simulink model "Exp_MLegMotor_PD_Sine"  (R2014b)
settings: Solver=ode1  StartTime=0.0  StopTime=Inf  FixedStep=0.001  RelTol=1e-3
PostLoadFcn:
  | , if any(exist('dsrtsu_mdlpostloadfcn', 'file') == [2, 3, 6]), try dsrtsu_mdlpostloadfcn('Execute', bdroot); catch fprintf('Error in PostLoadFcn (dsrtsu_mdlpostloadfcn) for model "%s":\n %s\n', bdroot, lasterr); end, end,
values from neighbouring files (symbols this model uses):
  coulomb_feedforward_coeff = 0    [init.m]
  enable_motor = 0    [init.m]
  filter_switch = 1    [init.m]
  Kd = 0.1    [init.m]
  Kp = 15    [init.m]
  motor_cutoff_angle = 70 * pi/180    (= 1.2217304764)    [init.m]
  motor_direction = -1    [init.m]
  pos_weight_1 = 0    [init.m]
  pos_weight_2 = 0    [init.m]
  ref_amplitude = 4    [init.m]
  ref_frequency = 0.5    [init.m]
  savgol_k = 2    [init.m]
  savgol_m = 150    [init.m]
  Ts = 0.001    [init.m]
undefined symbols (not defined in the file): max_ddphi, max_dphi, red_alpha, red_lambda
libraries: rtilib1103 x3, simulink x2, simulink_extras x1
settings Model: DSRTSU_INTERNAL_RTI_VER=450  DSRTSU_INTERNAL_RTI_TYPE=rti1103  DSRTSU_INTERNAL_RTIFPGA=40  TunableVars=Kd,Kp,coulomb_feedforward_coeff,enable_motor,filter_switch,motor_cutoff_angle,pos_weight_1,pos_weight_2,ref_amplitude,ref_frequency  TunableVarsStorageClass=Auto,Auto,Auto,Auto,Auto,Auto,Auto,Auto,Auto,Auto  TunableVarsTypeQualifier=,,,,,,,,,  BufferReuse=off  Creator=robotuser  LastModifiedBy=robotuser
settings OptimizationCC: BlockReduction=off  InlineParams=on  OptimizeBlockIOStorage=off  BufferReuse=off  GlobalBufferReuse=off  ExpressionFolding=off  LocalBlockOutputs=off
settings HardwareCC: ProdIntDivRoundTo=Zero  ProdEndianess=BigEndian  ProdHWDeviceType=Generic->Custom  TargetIntDivRoundTo=Zero  TargetEndianess=BigEndian  TargetHWDeviceType=Generic->Custom
settings RTWCC: SystemTargetFile=rti1103.tlc  MakeCommand=make_rti  TemplateMakefile=rti1103.tmf  Description=dSPACE DS1103 Hardware Platform  ProcessScript=rti1103_make_rtw_hook
settings STFCustomTargetCC: ParMdlRefBuildCompliant=on  GeneratePreprocessorConditionals=Disable all  SystemTargetFile=rti1103.tlc
settings GRTTargetCC: CompOptLevelCompliant=off  ConcurrentExecutionCompliant=off  CombineOutputUpdateFcns=off  MatFileLogging=off  CPPClassGenCompliant=off  GRTInterface=on  ExtModeMexFile=noextcomm

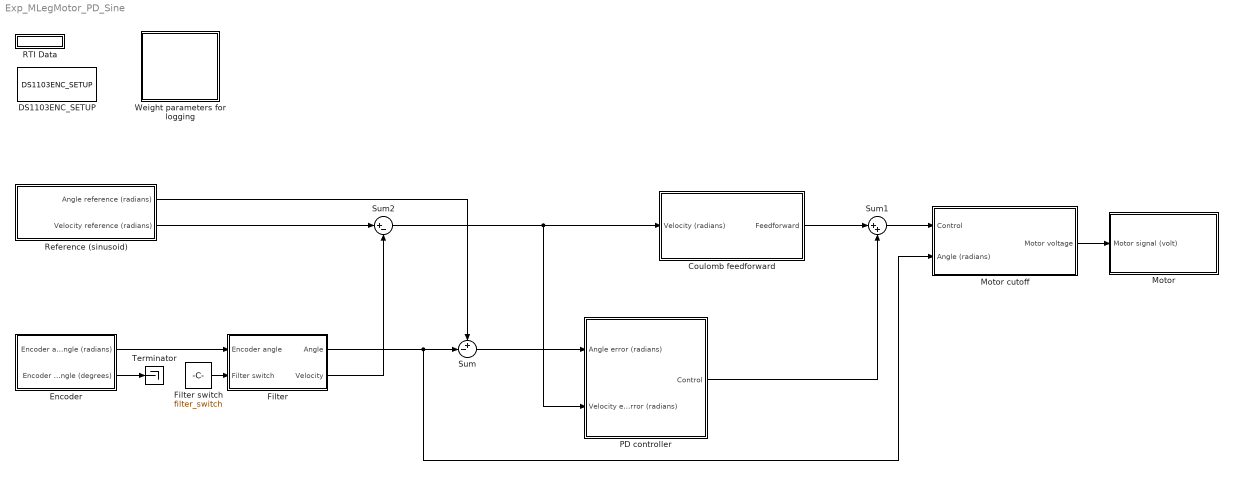
== system Exp_MLegMotor_PD_Sine ==
  Coulomb feedforward : Subsystem
  DS1103ENC_SETUP : rtilib1103/DS1103 MASTER PPC/DS1103ENC_SETUP  EncRange=0  Reserved1=[]  Reserved2=[]  Reserved3=[]  Reserved4=[]  DialogFcn=gui1103enc_setup  UnitName={ 'DS1103ENC_SETUP' }  UnitValues={ [] }  DSProperties=struct('RTI',struct('Version',uint32(1),'BlockType',struct('isSLSource',uint8(0),'isSLSink',uint8(0),'isHWSource',uint8(0),'isHWSink',uint8(0),'isSetup',uint8(0),'isInline',uint8(1),'isNonInline',uint8(0),'isInterrupt',uint8(0),'isChannelwise',uint8(0)),'IOBoardType','DS1103MASTER','UnitType','ENC','Identifier','ENCMASTER','DialogType','ML','BlockSet','NONE','SlaveProcessor','NONE'))
      settings: SignalType=[1 1 0 0 0 0 0]
  Encoder : Subsystem
  Filter : Subsystem
  Filter switch : Constant  Value=filter_switch
  Motor : Subsystem
  Motor cutoff : Subsystem
  PD controller : Subsystem  TreatAsAtomicUnit=on
  RTI Data : Subsystem  Tag=struct('RTIDataServer',struct('RTIDataServerVs','2','RTIModelDescription','struct(''main'',''Exp_MLegMotor_PD_Sine'',''sub'',''Exp_MLegMotor_PD_Sine'',''isMp'',0)'))  LoadFcn="if exist('rtidc'), try,  rtidc('DataHostBlockClbLoad', gcbh); catch, disp(['Warning: ''LoadFcn'' for RTI Data block failed: ' lasterr]); end, end,"  mask(RTI_DATA_HOST){}
      mask help:
      | RTI Data Block.
      | This block is used by RTI to store internal model-dependent data.
      | Please keep this block on the root level of the model. Deleting this block will result in data loss.
      |
      | NEVER DELETE OR COPY THIS BLOCK!
      settings: CopyFcn="if exist('rtidc'), try,  rtidc('DataHostBlockClbCopy', gcbh); catch, disp(['Warning: ''CopyFcn'' for RTI Data block failed: ' lasterr]); end, end,"  DeleteFcn="if exist('rtidc'), try,  rtidc('DataHostBlockClbDelete', gcbh); catch, disp(['Warning: ''DeleteFcn'' for RTI Data block failed: ' lasterr]); end, end,"  ModelCloseFcn="if exist('rtidc'), try,  rtidc('DataHostBlockClbModelClose', gcbh); catch, disp(['Warning: ''ModelCloseFcn'' for RTI Data block failed: ' lasterr]); end, end,"  PreSaveFcn="if exist('rtidc'), try,  rtidc('DataHostBlockClbPreSave', gcbh); catch, disp(['Warning: ''PreSaveFcn'' for RTI Data block failed: ' lasterr]); end, end,"  PostSaveFcn="if exist('rtidc'), try,  rtidc('DataHostBlockClbPostSave', gcbh); catch, disp(['Warning: ''PostSaveFcn'' for RTI Data block failed: ' lasterr]); end, end,"  NameChangeFcn="if exist('rtidc'), try,  rtidc('DataHostBlockClbNameChange', gcbh); catch, disp(['Warning: ''NameChangeFcn'' for RTI Data block failed: ' lasterr]); end, end,"
      mask Help:
      | RTI Data Block.
      | This block is used by RTI to store internal model-dependent data.
      | Please keep this block on the root level of the model. Deleting this block will result in data loss.
      | 
      | NEVER DELETE OR COPY THIS BLOCK!
      mask Display:
      | text(0.5, 0.5, 'RTI Data', 'HorizontalAlignment', 'center');
      | plot([1 0]);
  Reference (sinusoid) : Subsystem
  Sum : Sum  Inputs=+-|
  Sum1 : Sum  Inputs=|++
  Sum2 : Sum  Inputs=|+-
  Terminator : Terminator
  Weight parameters for logging : Subsystem
  wires:
  Coulomb feedforward/1(Feedforward) -> Sum1/1
  Encoder/1(Encoder angle (radians)) -> Filter/1(Encoder angle)
  Encoder/2(Encoder angle (degrees)) -> Terminator/1
  Reference (sinusoid)/1(Angle reference (radians)) -> Sum/1
  Reference (sinusoid)/2(Velocity reference (radians)) -> Sum2/1
  Filter/2(Velocity) -> Sum2/2
  Sum2/1 -> Coulomb feedforward/1(Velocity (radians)), PD controller/2(Velocity error (radians))
  Sum/1 -> PD controller/1(Angle error (radians))
  Filter switch/1 -> Filter/2(Filter switch)
  PD controller/1(Control) -> Sum1/2
  Filter/1(Angle) -> Motor cutoff/2(Angle (radians)), Sum/2
  Sum1/1 -> Motor cutoff/1(Control)
  Motor cutoff/1(Motor voltage) -> Motor/1(Motor signal (volt))

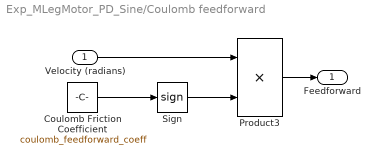
== system Exp_MLegMotor_PD_Sine/Coulomb feedforward ==
  Velocity (radians) : Inport
  Coulomb Friction Coefficient : Constant  Value=coulomb_feedforward_coeff
  Product3 : Product
  Sign : Signum
  Feedforward : Outport
  wires:
  Sign/1 -> Product3/2
  Velocity (radians)/1 -> Product3/1
  Product3/1 -> Feedforward/1
  Coulomb Friction Coefficient/1 -> Sign/1

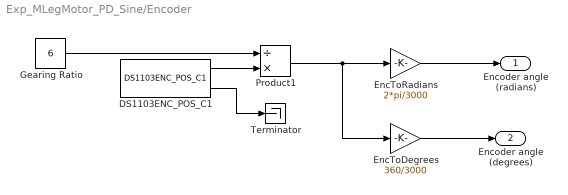
== system Exp_MLegMotor_PD_Sine/Encoder ==
  DS1103ENC_POS_C1 : rtilib1103/DS1103 MASTER PPC/DS1103ENC_POS_C1  ChannelNo=1  PosValue=0  Reserved1=[]  Reserved2=[]  Reserved3=[]  Reserved4=[]  DialogFcn=gui1103enc_pos  UnitName={ 'DS1103ENC_POS_C' }  UnitValues={1}  DSProperties=struct('RTI',struct('Version',uint32(1),'BlockType',struct('isSLSource',uint8(1),'isSLSink',uint8(0),'isHWSource',uint8(1),'isHWSink',uint8(0),'isSetup',uint8(0),'isInline',uint8(1),'isNonInline',uint8(0),'isInterrupt',uint8(0),'isChannelwise',uint8(1)),'IOBoardType','DS1103MASTER','UnitType','ENC','Identifier','ENCPOSCH','DialogType','ML','BlockSet','NONE','SlaveProcessor','NONE'))
  EncToDegrees : Gain  Gain=360/3000
  EncToRadians : Gain  Gain=2*pi/3000
  Gearing Ratio : Constant  Value=6
  Product1 : Product  Inputs=/*
  Terminator : Terminator
  Encoder angle (radians) : Outport
  Encoder angle (degrees) : Outport  Port=2
  wires:
  Product1/1 -> EncToDegrees/1, EncToRadians/1
  DS1103ENC_POS_C1/1 -> Product1/2
  Gearing Ratio/1 -> Product1/1
  DS1103ENC_POS_C1/2 -> Terminator/1
  EncToRadians/1 -> Encoder angle (radians)/1
  EncToDegrees/1 -> Encoder angle (degrees)/1

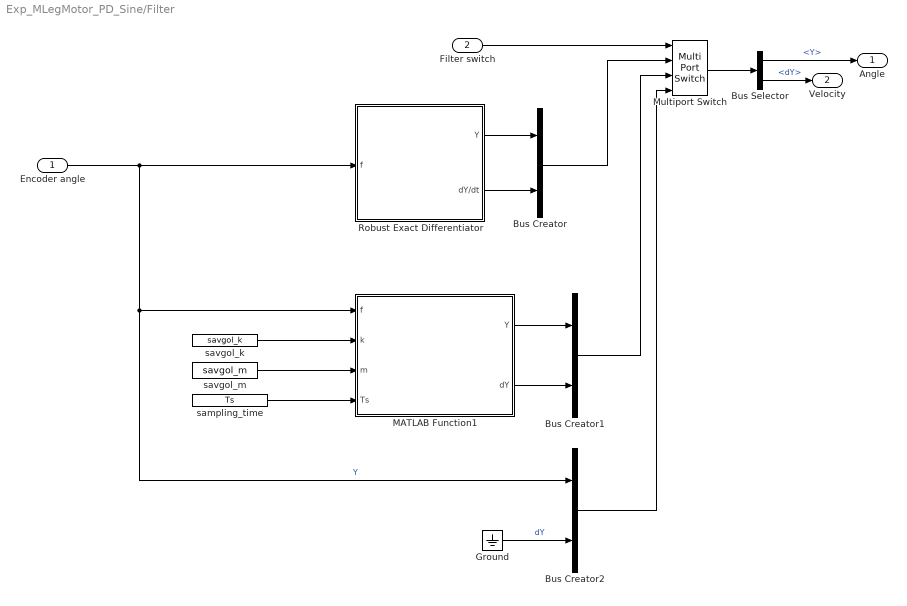
== system Exp_MLegMotor_PD_Sine/Filter ==
  Encoder angle : Inport
  Filter switch : Inport  Port=2
  Bus Creator : BusCreator  Inputs=2
  Bus Creator1 : BusCreator  Inputs=2
  Bus Creator2 : BusCreator  Inputs=2
  Bus Selector : BusSelector  OutputSignals=Y,dY
  Ground : Ground
  MATLAB Function1 : MATLAB Function  TreatAsAtomicUnit=on
  Multiport Switch : MultiPortSwitch
  Robust Exact Differentiator : Subsystem  mask{h=Ts, L=max_ddphi, M=max_dphi, lambda=red_lambda, alpha=red_alpha}
      mask prompts: h "h (sampling time)"; L "L = sup | d^2 f / dt^2 |"; M "M = sup | df /dt |"; lambda "lambda > 0"; alpha "alpha  > 0"
      mask Display:
      | port_label('output',1,' f(t)')
      | port_label('output',2,' df(t)/dt')
      | port_label('input',1,'f(t)+noise ')
  sampling_time : Constant  Value=Ts
  savgol_k : Constant  Value=savgol_k
  savgol_m : Constant  Value=savgol_m
  Angle : Outport
  Velocity : Outport  Port=2
  wires:
  savgol_k/1 -> MATLAB Function1/2(k)
  savgol_m/1 -> MATLAB Function1/3(m)
  sampling_time/1 -> MATLAB Function1/4(Ts)
  Encoder angle/1 -> Robust Exact Differentiator/1(f), Bus Creator2/1, MATLAB Function1/1(f)  "Y"
  Filter switch/1 -> Multiport Switch/1
  Multiport Switch/1 -> Bus Selector/1
  Bus Selector/1 -> Angle/1  "<Y>"
  Bus Selector/2 -> Velocity/1  "<dY>"
  Robust Exact Differentiator/1(Y) -> Bus Creator/1
  Robust Exact Differentiator/2(dY/dt) -> Bus Creator/2
  Bus Creator/1 -> Multiport Switch/2
  MATLAB Function1/1(Y) -> Bus Creator1/1
  MATLAB Function1/2(dY) -> Bus Creator1/2
  Bus Creator1/1 -> Multiport Switch/3
  Ground/1 -> Bus Creator2/2  "dY"
  Bus Creator2/1 -> Multiport Switch/4

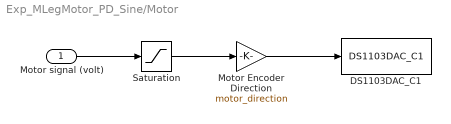
== system Exp_MLegMotor_PD_Sine/Motor ==
  Motor signal (volt) : Inport
  DS1103DAC_C1 : rtilib1103/DS1103 MASTER PPC/DS1103DAC_C1  ChannelNo=1  InitValue=0  TermMode=1  TermValue=0  Reserved1=[]  Reserved2=[]  Reserved3=[]  Reserved4=[]  DialogFcn=gui1103dac  UnitName={ 'DS1103DAC_C' }  UnitValues={ 1 }  DSProperties=struct('RTI',struct('Version',uint32(1),'BlockType',struct('isSLSource',uint8(0),'isSLSink',uint8(1),'isHWSource',uint8(0),'isHWSink',uint8(1),'isSetup',uint8(0),'isInline',uint8(1),'isNonInline',uint8(0),'isInterrupt',uint8(0),'isChannelwise',uint8(1)),'IOBoardType','DS1103MASTER','UnitType','DAC','Identifier','DAC','DialogType','ML','BlockSet','NONE','SlaveProcessor','NONE'))
  "Motor Encoder Direction " : Gain  Gain=motor_direction
  Saturation : Saturate  UpperLimit=10  LowerLimit=-10
  wires:
  Saturation/1 -> "Motor Encoder Direction "/1
  "Motor Encoder Direction "/1 -> DS1103DAC_C1/1
  Motor signal (volt)/1 -> Saturation/1

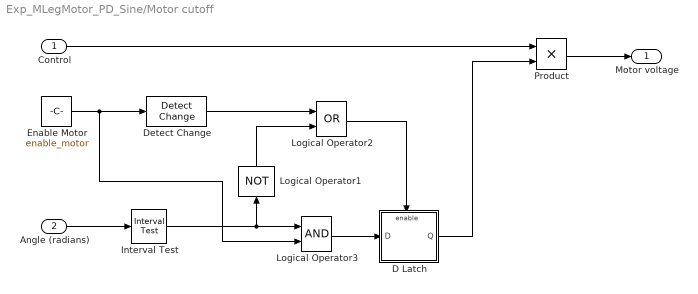
== system Exp_MLegMotor_PD_Sine/Motor cutoff ==
  Control : Inport
  Angle (radians) : Inport  Port=2
  D Latch : Subsystem
  Detect Change : simulink/Logic and Bit Operations/Detect Change  vinit=0  InputProcessing=Inherited  OutDataTypeStr=boolean
  Enable Motor : Constant  Value=enable_motor  OutDataTypeStr=boolean
  Interval Test : simulink/Logic and Bit Operations/Interval Test  IntervalClosedRight=on  uplimit=motor_cutoff_angle  IntervalClosedLeft=on  lowlimit=-motor_cutoff_angle  OutDataTypeStr=boolean
  Logical Operator1 : Logic  Operator=NOT  AllPortsSameDT=off  OutDataTypeStr=boolean
  Logical Operator2 : Logic  Operator=OR  AllPortsSameDT=off  OutDataTypeStr=boolean
  Logical Operator3 : Logic  AllPortsSameDT=off  OutDataTypeStr=boolean
  Product : Product
  Motor voltage : Outport
  wires:
  Enable Motor/1 -> Detect Change/1, Logical Operator3/2
  Interval Test/1 -> Logical Operator3/1, Logical Operator1/1
  Angle (radians)/1 -> Interval Test/1
  Detect Change/1 -> Logical Operator2/1
  Logical Operator2/1 -> D Latch/Enable
  Logical Operator1/1 -> Logical Operator2/2
  Logical Operator3/1 -> D Latch/1(D)
  D Latch/1(Q) -> Product/2
  Product/1 -> Motor voltage/1
  Control/1 -> Product/1

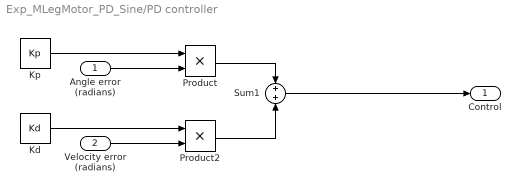
== system Exp_MLegMotor_PD_Sine/PD controller ==
  Angle error (radians) : Inport
  Velocity error (radians) : Inport  Port=2
  Kd : Constant  Value=Kd
  Kp : Constant  Value=Kp
  Product : Product
  Product2 : Product
  Sum1 : Sum  Inputs=+|+
  Control : Outport
  wires:
  Angle error (radians)/1 -> Product/2
  Kp/1 -> Product/1
  Kd/1 -> Product2/1
  Product2/1 -> Sum1/2
  Product/1 -> Sum1/1
  Velocity error (radians)/1 -> Product2/2
  Sum1/1 -> Control/1

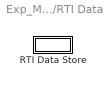
== system Exp_MLegMotor_PD_Sine/RTI Data ==
  RTI Data Store : Subsystem  Tag=struct('private',struct('version',struct('dsVer',uint32(2)),'access',struct('modified',['24-Mar-2017 15:05:46'],'type','Model','isPerm',1)))  mask(RTI_DATA_STORE){}
      mask help:
      | RTI Data Store Block. This block is used by RTI to store internal model dependent data. Deleting this block will result in data loss.
      |
      | NEVER DELETE, COPY, OR MODIFY THIS BLOCK!
      mask Help:
      | RTI Data Store Block. This block is used by RTI to store internal model dependent data. Deleting this block will result in data loss.
      | 
      | NEVER DELETE, COPY, OR MODIFY THIS BLOCK!
      mask Display: text(0.5, 0.5, ' ', 'HorizontalAlignment', 'center');

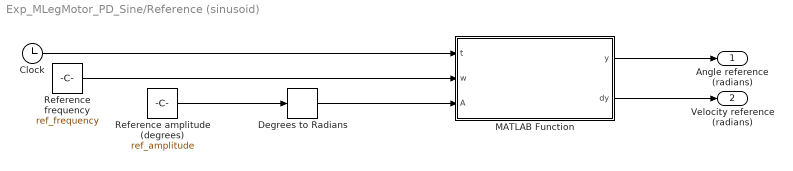
== system Exp_MLegMotor_PD_Sine/Reference (sinusoid) ==
  Clock : Clock
  Degrees to Radians : simulink_extras/Transformations/Degrees to Radians
  MATLAB Function : MATLAB Function  TreatAsAtomicUnit=on
  Reference amplitude (degrees) : Constant  Value=ref_amplitude
  Reference frequency : Constant  Value=ref_frequency
  Angle reference (radians) : Outport
  Velocity reference (radians) : Outport  Port=2
  wires:
  Clock/1 -> MATLAB Function/1(t)
  Reference frequency/1 -> MATLAB Function/2(w)
  MATLAB Function/1(y) -> Angle reference (radians)/1
  MATLAB Function/2(dy) -> Velocity reference (radians)/1
  Reference amplitude (degrees)/1 -> Degrees to Radians/1
  Degrees to Radians/1 -> MATLAB Function/3(A)

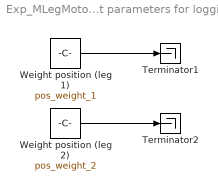
== system Exp_MLegMotor_PD_Sine/Weight parameters for logging ==
  Terminator1 : Terminator
  Terminator2 : Terminator
  Weight position (leg 1) : Constant  Value=pos_weight_1
  Weight position (leg 2) : Constant  Value=pos_weight_2
  wires:
  Weight position (leg 2)/1 -> Terminator2/1
  Weight position (leg 1)/1 -> Terminator1/1

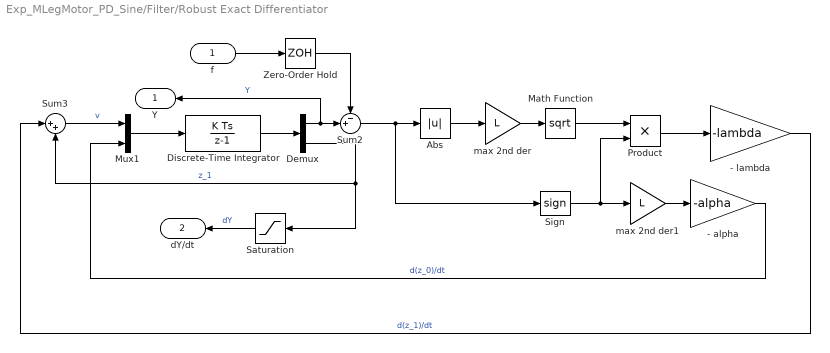
== system Exp_MLegMotor_PD_Sine/Filter/Robust Exact Differentiator ==
  f : Inport
  - alpha : Gain  Gain=-alpha
  - lambda : Gain  Gain=-lambda
  Abs : Abs  ZeroCross=off
  Demux : Demux  Outputs=2
  Discrete-Time Integrator : DiscreteIntegrator  InitialCondition=[0 0]  SampleTime=h
  Math Function : Math  Operator=sqrt  SaturateOnIntegerOverflow=on
  Mux1 : Mux  Inputs=2
  Product : Product  RndMeth=Zero
  Saturation : Saturate  UpperLimit=M  LowerLimit=-M
  Sign : Signum  ZeroCross=off
  Sum2 : Sum  Inputs=-+|
  Sum3 : Sum  Inputs=|++
  Zero-Order Hold : ZeroOrderHold  SampleTime=h
  max 2nd der : Gain  Gain=L
  max 2nd der1 : Gain  Gain=L
  Y : Outport
  dY/dt : Outport  Port=2
  wires:
  Zero-Order Hold/1 -> Sum2/1
  f/1 -> Zero-Order Hold/1
  max 2nd der1/1 -> - alpha/1
  max 2nd der/1 -> Math Function/1
  - lambda/1 -> Sum3/1  "d(z_1)/dt"
  Product/1 -> - lambda/1
  Abs/1 -> max 2nd der/1
  Sum3/1 -> Mux1/1  "v"
  - alpha/1 -> Mux1/2  "d(z_0)/dt"
  Sign/1 -> max 2nd der1/1, Product/2
  Sum2/1 -> Abs/1, Sign/1
  Mux1/1 -> Discrete-Time Integrator/1
  Discrete-Time Integrator/1 -> Demux/1
  Demux/1 -> Y/1, Sum2/2  "Y"
  Demux/2 -> Sum3/2, Saturation/1  "z_1"
  Math Function/1 -> Product/1
  Saturation/1 -> dY/dt/1  "dY"

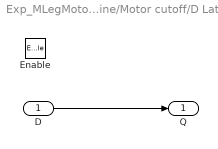
== system Exp_MLegMotor_PD_Sine/Motor cutoff/D Latch ==
  D : Inport
  Enable : EnablePort
  Q : Outport
  wires:
  D/1 -> Q/1

== system Exp_MLegMotor_PD_Sine/RTI Data/RTI Data Store ==
  RTI Data Store : Subsystem  mask(RTI_DATA_STORE){}
      mask help:
      | RTI Data Store Block. This block is used by RTI to store internal model dependent data. Deleting this block will result in data loss.
      |
      | NEVER DELETE, COPY, OR MODIFY THIS BLOCK!
      mask Help:
      | RTI Data Store Block. This block is used by RTI to store internal model dependent data. Deleting this block will result in data loss.
      | 
      | NEVER DELETE, COPY, OR MODIFY THIS BLOCK!
      mask Display: text(0.5, 0.5, ' ', 'HorizontalAlignment', 'center');

== system Exp_MLegMotor_PD_Sine/RTI Data/RTI Data Store/RTI Data Store ==
  RTI Data Store : Subsystem  mask(RTI_DATA_STORE){}
      mask help:
      | RTI Data Store Block. This block is used by RTI to store internal model dependent data. Deleting this block will result in data loss.
      |
      | NEVER DELETE, COPY, OR MODIFY THIS BLOCK!
      mask Help:
      | RTI Data Store Block. This block is used by RTI to store internal model dependent data. Deleting this block will result in data loss.
      | 
      | NEVER DELETE, COPY, OR MODIFY THIS BLOCK!
      mask Display: text(0.5, 0.5, ' ', 'HorizontalAlignment', 'center');

== system Exp_MLegMotor_PD_Sine/RTI Data/RTI Data Store/RTI Data Store/RTI Data Store ==
  RTI Data Store : Subsystem  mask(RTI_DATA_STORE){}
      mask help:
      | RTI Data Store Block. This block is used by RTI to store internal model dependent data. Deleting this block will result in data loss.
      |
      | NEVER DELETE, COPY, OR MODIFY THIS BLOCK!
      mask Help:
      | RTI Data Store Block. This block is used by RTI to store internal model dependent data. Deleting this block will result in data loss.
      | 
      | NEVER DELETE, COPY, OR MODIFY THIS BLOCK!
      mask Display: text(0.5, 0.5, ' ', 'HorizontalAlignment', 'center');

== system Exp_MLegMotor_PD_Sine/RTI Data/RTI Data Store/RTI Data Store/RTI Data Store/RTI Data Store ==

== matlab function Exp_MLegMotor_PD_Sine/Filter/MATLAB Function1 ==
  data: f input; Y output; dY output; k input; m input; Ts input
function [Y, dY] = savgol(f, k, m, Ts)
    assert(k < 10);
    assert(m < 1000);
    assert(Ts < 1);
    [Y, dY] = savgol_filter(f, k, m, Ts);

== matlab function Exp_MLegMotor_PD_Sine/Reference (sinusoid)/MATLAB Function ==
  data: t input; y output; w input; A input; dy output
function [y, dy] = sine(t, w, A)
    [y, dy] = cont_sine(t, w, A);
